simulink model "timeDomainFeaturesTest"  (R2020b)
settings: Solver=FixedStepDiscrete  StartTime=0.0  StopTime=stopTime  RelTol=1e-3
PostLoadFcn:
  | addpath([fileparts(which(bdroot)) filesep '..' filesep])
  | loadDataSimulinkCallback
InitFcn:
  | simulinkInitTimeDomainFeatures
StopFcn:
  | simulinkVerifyTimeDomainFeatures
undefined symbols (not defined in the file or in its folder): params
libraries: dspsrcs4 x1
settings Model: DataTypeOverride=Off  SimulationMode=accelerator  PauseTimes=1  Creator=trevor  LastModifiedBy=trevor
settings DataIOCC: SaveFormat=Array  SaveOutput=off  DSMLogging=off  SaveTime=off  ReturnWorkspaceOutputs=off
settings OptimizationCC: BlockReduction=off  ConditionallyExecuteInputs=off  DefaultParameterBehavior=Inlined
settings DebuggingCC: SignalRangeChecking=warning  AlgebraicLoopMsg=error  SingleTaskRateTransMsg=error  SFMachineParentedDataDiag=error
settings HardwareCC: ProdBitPerPointer=32  ProdBitPerSizeT=32  ProdBitPerPtrDiffT=32  ProdLargestAtomicFloat=None  ProdIntDivRoundTo=Undefined  ProdEndianess=Unspecified  ProdWordSize=32  ProdHWDeviceType=ASIC/FPGA->ASIC/FPGA  TargetBitPerLong=64  TargetBitPerPointer=64  TargetBitPerSizeT=64  TargetBitPerPtrDiffT=64  TargetLongLongMode=on  TargetIntDivRoundTo=Zero  TargetEndianess=LittleEndian  TargetWordSize=64  TargetHWDeviceType=Custom Processor->MATLAB Host Computer  ProdEqTarget=off
settings SFSimCC: SFSimEcho=off

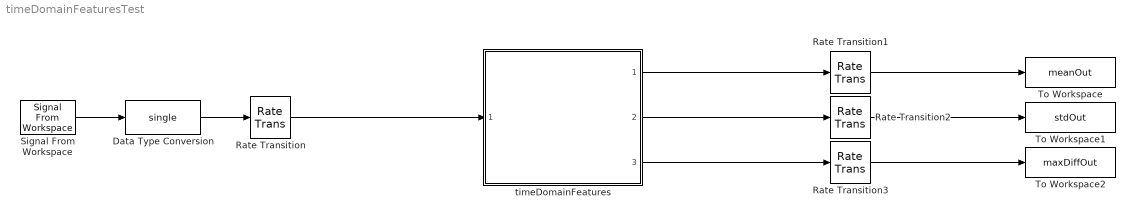
== system timeDomainFeaturesTest ==
  Data Type Conversion : DataTypeConversion  OutDataTypeStr=single
  Rate Transition : RateTransition  OutPortSampleTime=params.systemClockPeriod
  Rate Transition1 : RateTransition  OutPortSampleTime=params.samplingPeriod
  Rate Transition2 : RateTransition  OutPortSampleTime=params.samplingPeriod
  Rate Transition3 : RateTransition  OutPortSampleTime=params.samplingPeriod
  Signal From Workspace : dspsrcs4/Signal From Workspace  X=testData  Ts=params.samplingPeriod  nsamps=1  OutputAfterFinalValue=Setting to zero  ignoreOrWarnInputAndFrameLengths=off  OutputFrames=off
  To Workspace : ToWorkspace  VariableName=meanOut  SampleTime=-1
      settings: Save2DSignal=2-D array (concatenate along first dimension)
  To Workspace1 : ToWorkspace  VariableName=stdOut  SampleTime=-1
      settings: Save2DSignal=2-D array (concatenate along first dimension)
  To Workspace2 : ToWorkspace  VariableName=maxDiffOut  SampleTime=-1
      settings: Save2DSignal=2-D array (concatenate along first dimension)
  timeDomainFeatures : Subsystem  ReferencedSubsystem=timeDomainFeatures
  wires:
  timeDomainFeatures/1 -> Rate Transition1/1
  timeDomainFeatures/2 -> Rate Transition2/1
  timeDomainFeatures/3 -> Rate Transition3/1
  Rate Transition/1 -> timeDomainFeatures/1
  Rate Transition1/1 -> To Workspace/1
  Rate Transition2/1 -> To Workspace1/1
  Rate Transition3/1 -> To Workspace2/1
  Signal From Workspace/1 -> Data Type Conversion/1
  Data Type Conversion/1 -> Rate Transition/1
